simulink model "optimal_servo_control"  (R2016a)
settings: Solver=ode4  StartTime=0.0  StopTime=1  RelTol=1e-3
settings Model: Creator=shohei  LastModifiedBy=shohei

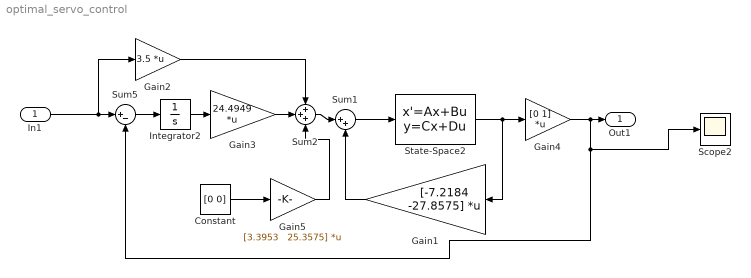
== system optimal_servo_control ==
  In1 : Inport
  Constant : Constant  Value=[0 0]
  Gain1 : Gain  Gain=[-7.2184 -27.8575]  Multiplication=Matrix(K*u)
  Gain2 : Gain  Gain=3.5  Multiplication=Matrix(K*u)
  Gain3 : Gain  Gain=24.4949  Multiplication=Matrix(K*u)
  Gain4 : Gain  Gain=[0 1]  Multiplication=Matrix(K*u)
  Gain5 : Gain  Gain="[3.3953   25.3575]"  Multiplication=Matrix(K*u)
  Integrator2 : Integrator
  Scope2 : Scope
  State-Space2 : StateSpace  A=[-0.125 -0.5; 0.5 0]  B=[0.5;0]  C=eye(2)  D=[0;0]  X0=0
  Sum1 : Sum  Inputs=|++
  Sum2 : Sum  Inputs=+++
  Sum5 : Sum  Inputs=|+-
  Out1 : Outport
  wires:
  State-Space2/1 -> Gain1/1, Gain4/1
  In1/1 -> Gain2/1, Sum5/1
  Sum5/1 -> Integrator2/1
  Integrator2/1 -> Gain3/1
  Gain2/1 -> Sum2/1
  Sum2/1 -> Sum1/1
  Gain1/1 -> Sum1/2
  Sum1/1 -> State-Space2/1
  Gain3/1 -> Sum2/2
  Constant/1 -> Gain5/1
  Gain5/1 -> Sum2/3
  Gain4/1 -> Out1/1, Scope2/1, Sum5/2
